simulink model "prison_rf_sensor_localisation_model"  (R2024b)
settings: Solver=FixedStepDiscrete  StartTime=0.0  StopTime=116  FixedStep=1  RelTol=1e-3
settings Model: Creator=pnaga  LastModifiedBy=pnaga

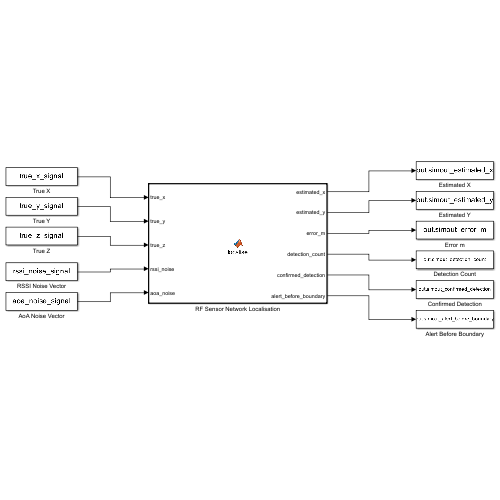
[thumbnail: Simulink's stored preview of the top-level diagram]
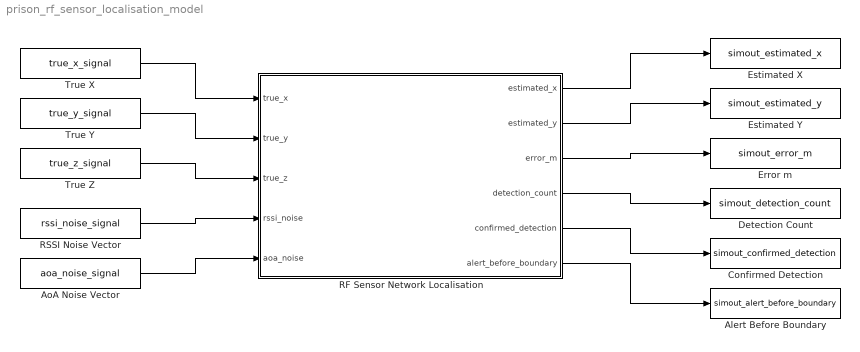
== system prison_rf_sensor_localisation_model ==
  Alert Before Boundary : ToWorkspace  VariableName=simout_alert_before_boundary  SaveFormat=Timeseries  SampleTime=-1
  AoA Noise Vector : FromWorkspace  VariableName=aoa_noise_signal
  Confirmed Detection : ToWorkspace  VariableName=simout_confirmed_detection  SaveFormat=Timeseries  SampleTime=-1
  Detection Count : ToWorkspace  VariableName=simout_detection_count  SaveFormat=Timeseries  SampleTime=-1
  Error m : ToWorkspace  VariableName=simout_error_m  SaveFormat=Timeseries  SampleTime=-1
  Estimated X : ToWorkspace  VariableName=simout_estimated_x  SaveFormat=Timeseries  SampleTime=-1
  Estimated Y : ToWorkspace  VariableName=simout_estimated_y  SaveFormat=Timeseries  SampleTime=-1
  RF Sensor Network Localisation : MATLAB Function  TreatAsAtomicUnit=on
  RSSI Noise Vector : FromWorkspace  VariableName=rssi_noise_signal
  True X : FromWorkspace  VariableName=true_x_signal
  True Y : FromWorkspace  VariableName=true_y_signal
  True Z : FromWorkspace  VariableName=true_z_signal
  wires:
  True X/1 -> RF Sensor Network Localisation/1(true_x)
  True Y/1 -> RF Sensor Network Localisation/2(true_y)
  True Z/1 -> RF Sensor Network Localisation/3(true_z)
  RSSI Noise Vector/1 -> RF Sensor Network Localisation/4(rssi_noise)
  AoA Noise Vector/1 -> RF Sensor Network Localisation/5(aoa_noise)
  RF Sensor Network Localisation/1(estimated_x) -> Estimated X/1
  RF Sensor Network Localisation/2(estimated_y) -> Estimated Y/1
  RF Sensor Network Localisation/3(error_m) -> Error m/1
  RF Sensor Network Localisation/4(detection_count) -> Detection Count/1
  RF Sensor Network Localisation/5(confirmed_detection) -> Confirmed Detection/1
  RF Sensor Network Localisation/6(alert_before_boundary) -> Alert Before Boundary/1

== matlab function prison_rf_sensor_localisation_model/RF Sensor Network Localisation ==
  data: true_x input; estimated_x output; true_y input; true_z input; rssi_noise input; aoa_noise input; estimated_y output; error_m output; detection_count output; confirmed_detection output; alert_before_boundary output
function [estimated_x, estimated_y, error_m, detection_count, confirmed_detection, alert_before_boundary] = localise(true_x, true_y, true_z, rssi_noise, aoa_noise)
%#codegen
sensorX = [250;250;250;250;250;250;300;400;600;700;750;750;750;750;750;750;700;600;400;300;300;500;700;500];
sensorY = [300;350;450;550;650;700;700;700;700;700;700;650;550;450;350;300;300;300;300;300;500;350;500;650];
sensorZ = 15 * ones(24,1);
orientation = atan2d(sensorY - 500, sensorX - 500);
fov = 120 * ones(24,1);
threshold = -65 * ones(24,1);
frequencyHz = 2.4e9;
txPowerDbm = 20;
txGainDbi = 0;
rxGainDbi = 0;
rssiSigmaDb = 1;
aoaSigmaDeg = 0.5;
rxNoisy = zeros(24,1);
measuredBearing = zeros(24,1);
detected = false(24,1);
detection_count = 0;
for s = 1:24
    dx = true_x - sensorX(s);
    dy = true_y - sensorY(s);
    dz = true_z - sensorZ(s);
    distance = max(sqrt(dx*dx + dy*dy + dz*dz), 1);
    pathLossDb = 20 * log10(distance) + 20 * log10(frequencyHz) - 147.55;
    rxIdeal = txPowerDbm + txGainDbi + rxGainDbi - pathLossDb;
    rxNoisy(s) = rxIdeal + rssi_noise(s);
    trueBearing = atan2d(dy, dx);
    measuredBearing(s) = wrap180Local(trueBearing + aoa_noise(s));
    angleFromBoresight = wrap180Local(trueBearing - orientation(s));
    detected(s) = abs(angleFromBoresight) <= fov(s)/2 && rxNoisy(s) >= threshold(s);
    if detected(s)
        detection_count = detection_count + 1;
    end
end
confirmed_detection = double(detection_count >= 2);
outsideSecureWall = true_x < 300 || true_x > 700 || true_y < 350 || true_y > 650;
alert_before_boundary = double(confirmed_detection > 0 && outsideSecureWall);
estimated_x = NaN;
estimated_y = NaN;
error_m = NaN;
if detection_count < 2
    return;
end
sensorXd = zeros(24,1); sensorYd = zeros(24,1); ranges = zeros(24,1); bearingsRad = zeros(24,1); rangeStd = zeros(24,1);
n = 0;
for s = 1:24
    if detected(s)
        n = n + 1;
        sensorXd(n) = sensorX(s);
        sensorYd(n) = sensorY(s);
        ranges(n) = 10^((txPowerDbm + txGainDbi + rxGainDbi - rxNoisy(s) - 20*log10(frequencyHz) + 147.55)/20);
        bearingsRad(n) = measuredBearing(s) * pi / 180;
        rangeStd(n) = max((log(10)/20) * rssiSigmaDb * ranges(n), 1);
    end
end
pos = [0; 0];
for i = 1:n
    pos(1) = pos(1) + sensorXd(i) + ranges(i) * cos(bearingsRad(i));
    pos(2) = pos(2) + sensorYd(i) + ranges(i) * sin(bearingsRad(i));
end
pos = pos / n;
bearingStd = max(aoaSigmaDeg, 0.1) * pi / 180;
for iter = 1:25
    H = zeros(2,2);
    g = zeros(2,1);
    for i = 1:n
        dx = pos(1) - sensorXd(i);
        dy = pos(2) - sensorYd(i);
        predictedRange = max(sqrt(dx*dx + dy*dy), 1e-6);
        predictedBearing = atan2(dy, dx);
        rr = predictedRange - ranges(i);
        Jr = [dx/predictedRange, dy/predictedRange];
        wr = 1 / rangeStd(i);
        rb = wrapPiLocal(predictedBearing - bearingsRad(i));
        Jb = [-dy/(predictedRange*predictedRange), dx/(predictedRange*predictedRange)];
        wb = 1 / bearingStd;
        H = H + (Jr' * Jr) * wr * wr + (Jb' * Jb) * wb * wb;
        g = g + Jr' * rr * wr * wr + Jb' * rb * wb * wb;
    end
    step = -((H + 1e-5 * eye(2)) \ g);
    pos = pos + step;
    if sqrt(step(1)*step(1) + step(2)*step(2)) < 1e-4
        break;
    end
end
estimated_x = pos(1);
estimated_y = pos(2);
error_m = sqrt((estimated_x - true_x)^2 + (estimated_y - true_y)^2);
end
function angle = wrap180Local(angle)
angle = mod(angle + 180, 360) - 180;
end
function angle = wrapPiLocal(angle)
angle = mod(angle + pi, 2*pi) - pi;
end
